simulink model "untitled4b"  (Simulink 3.00)
settings: Solver=ode45  StartTime=0.0  StopTime=3  RelTol=1e-3

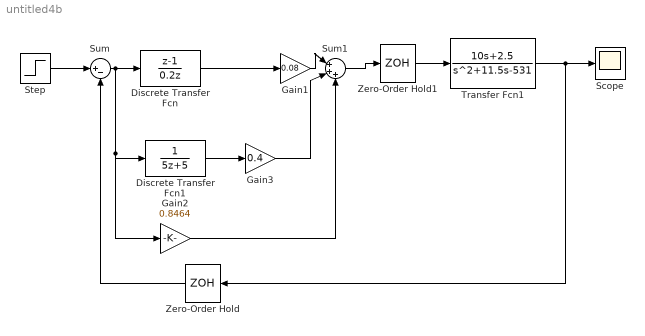
== system untitled4b ==
  Discrete Transfer Fcn : DiscreteTransferFcn  Numerator=[1 -1]  Denominator=[0.2 0]  SampleTime=0.25
  Discrete Transfer Fcn1 : DiscreteTransferFcn  Numerator=[1]  Denominator=[5 5]  SampleTime=1
  Gain1 : Gain  Gain=0.08  SaturateOnIntegerOverflow=on
  Gain2 : Gain  Gain=0.8464  SaturateOnIntegerOverflow=on
  Gain3 : Gain  Gain=0.4  SaturateOnIntegerOverflow=on
  Scope : Scope
      settings: TimeRange=10  YMin=-3e+024  YMax=1e+024  SaveToWorkspace=off  SaveName=ScopeData
  Step : Step  Time=0  Before=0  After=1  SampleTime=0
  Sum : Sum  Inputs=|+-  SaturateOnIntegerOverflow=on
  Sum1 : Sum  Inputs=|+++  SaturateOnIntegerOverflow=on
  Transfer Fcn1 : TransferFcn  Numerator=[10 2.5]  Denominator=[1 11.5 -531]
  Zero-Order Hold : ZeroOrderHold  Orientation=left  SampleTime=0.2
  Zero-Order Hold1 : ZeroOrderHold  SampleTime=0.2
  wires:
  Zero-Order Hold1/1 -> Transfer Fcn1/1
  Zero-Order Hold/1 -> Sum/2
  Step/1 -> Sum/1
  Transfer Fcn1/1 -> Scope/1, Zero-Order Hold/1
  Gain1/1 -> Sum1/1
  Discrete Transfer Fcn/1 -> Gain1/1
  Sum/1 -> Discrete Transfer Fcn/1, Discrete Transfer Fcn1/1, Gain2/1
  Discrete Transfer Fcn1/1 -> Gain3/1
  Gain3/1 -> Sum1/2
  Gain2/1 -> Sum1/3
  Sum1/1 -> Zero-Order Hold1/1
